simulink model "Yd1"  (R2021a)
settings: Solver=ode5  StartTime=0.0  StopTime=0.02  FixedStep=2e-6  RelTol=1e-3
InitFcn:
  | Pn = 3000;
  | fg = 50;
  | 
  | Vp = 440;
  | Vs = 220;
  | rp = 100e-3;
  | Lp = 3.5e-3;
  | Rc = 1500;
  | Lm = 1500e-3;
undefined symbols (not defined in the file): Lo_act, ro_act, Vo
libraries: spsLinearTransformerLib x3, dspstat3 x2, spsVoltageMeasurementLib x2, spsThreePhaseProgrammableVoltageSourceLib x1, spspowerguiLib x1
settings Model: Creator=Triptendu  LastModifiedBy=mansi
settings SolverCC: AlgebraicLoopSolver=TrustRegion
settings DebuggingCC: SFMachineParentedDataDiag=warning

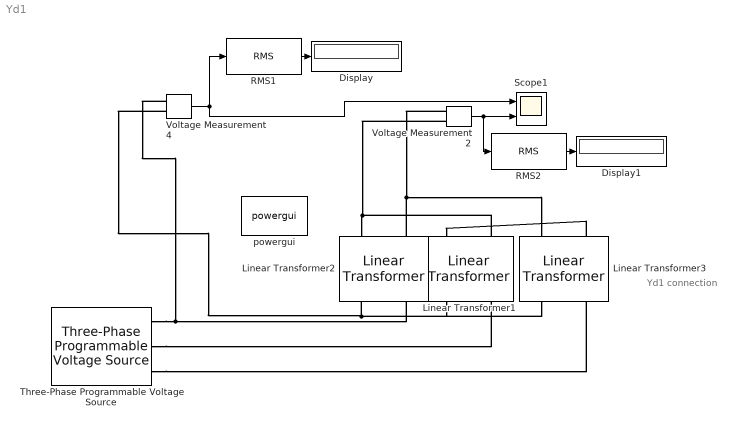
== system Yd1 ==
  note: Yd1 connection
  Display : Display
  Display1 : Display
  Linear Transformer1 : spsLinearTransformerLib/Linear Transformer  UNITS=SI  NominalPower=[3000 50]  winding1=[440 0.1 0.0035]  winding2=[220 1e-6 0]  ThreeWindings=off  winding3=[Vo/2 ro_act/2 Lo_act/2]  RmLm=[1500 1.5]  Measurements=None  DataType=on
  Linear Transformer2 : spsLinearTransformerLib/Linear Transformer  UNITS=SI  NominalPower=[3000 50]  winding1=[440 0.1 0.0035]  winding2=[220 1e-6 0]  ThreeWindings=off  winding3=[Vo/2 ro_act/2 Lo_act/2]  RmLm=[1500 1.5]  Measurements=None  DataType=on
  Linear Transformer3 : spsLinearTransformerLib/Linear Transformer  UNITS=SI  NominalPower=[3000 50]  winding1=[440 0.1 0.0035]  winding2=[220 1e-6 0]  ThreeWindings=off  winding3=[Vo/2 ro_act/2 Lo_act/2]  RmLm=[1500 1.5]  Measurements=None  DataType=on
  RMS1 : dspstat3/RMS  run=off  directionMode=Each column  dimension=1  InputProcessing=Columns as channels (frame based)  reset_popup=None
  RMS2 : dspstat3/RMS  run=off  directionMode=Each column  dimension=1  InputProcessing=Columns as channels (frame based)  reset_popup=None
  Scope1 : Scope  NumInputPorts=2
  Three-Phase Programmable Voltage Source : spsThreePhaseProgrammableVoltageSourceLib/Three-Phase Programmable Voltage Source  PositiveSequence="[440  0 50]"  VariationEntity=None  VariationType=Table of time-amplitude pairs  VariationTypeAlt=Step  VariationStep=0.5  VariationRate=10  VariationMagnitude=0.3  VariationFrequency=2  VariationTiming=[1 2]  VariationPhaseA=off  Amplitudes=[1 0.8 1.2 1.0]  TimeValues=[0 0.1 0.15 0.2]  HarmonicGeneration=off  HarmonicA=[3 0.2 -25 0]  HarmonicB=[2 0.15 35 2]  Timing="[0.05  3]"  BusType=swing  Pref=0  Qref=0  Qmin=-inf  Qmax=inf
  Voltage Measurement2 : spsVoltageMeasurementLib/Voltage Measurement  PhasorSimulation=off  OutputType=Complex  PSBequivalent=0
  Voltage Measurement4 : spsVoltageMeasurementLib/Voltage Measurement  PhasorSimulation=off  OutputType=Complex  PSBequivalent=0
  powergui : spspowerguiLib/powergui  Priority=1  SimulationMode=Discrete  SampleTime=2e-6  frequency=60  Iterations=50  frequencyindice=50  Pbase=100e6  ErrMax=1e-4  UnitsV=kV  UnitsW=MW  buscounter=0  FunctionMessages=off  echomessages=off  EnableUseOfTLC=off  CurrentSourceSwitches=off  DisableSnubberDevices=off  DisableRonSwitches=off  DisableVfSwitches=off  DisplayEquations=off  AutomaticDiscreteSolvers=off  SolverType=Backward Euler  Interpol=off  ExternalGateDelay=off  methode=off  Ts=100  x0status=blocks  SPID=on  SwTol=0  HookPort=off  NonlinearTolerance=1e-4  nMaxIteration=100  ContinueOnMaxIteration=off  RestoreLinks=warning  ResistiveCurrentMeasurement=off  Frange=[0:2:500]  Ylog=off  Xlog=on  ShowGrid=off  save=off  variable=ZData  structure=0  ZoomFFT=off  StartTime=0.0  cycles=1  DisplayStyle=1  fundamental=60  FreqAxis=off  MaxFrequency=1000  frequencyindicesteady=1  RmsSteady=1  display=off
  wires:
  RMS1/1 -> Display/1
  Voltage Measurement4/1 -> Scope1/1, RMS1/1
  Voltage Measurement2/1 -> RMS2/1, Scope1/2
  RMS2/1 -> Display1/1
  connections:
  Linear Transformer3/RConn1 -- Linear Transformer1/RConn2
  Linear Transformer1/RConn1 -- Voltage Measurement2/LConn2 -- Linear Transformer2/RConn2
  Linear Transformer2/RConn1 -- Voltage Measurement2/LConn1 -- Linear Transformer3/RConn2
  Three-Phase Programmable Voltage Source/RConn1 -- Voltage Measurement4/LConn1 -- Linear Transformer2/LConn1
  Three-Phase Programmable Voltage Source/RConn2 -- Linear Transformer1/LConn1
  Three-Phase Programmable Voltage Source/RConn3 -- Linear Transformer3/LConn1
  Voltage Measurement4/LConn2 -- Linear Transformer3/LConn2 -- Linear Transformer1/LConn2 -- Linear Transformer2/LConn2
